simulink model "DC_Simscape_test_Sem_Graph"  (R2016a)
settings: Solver=ode15s  StartTime=0.0  StopTime=20  RelTol=1e-3
PreLoadFcn:
  | t_sim = 1;
  | T = 25;
libraries: fl_lib x16, nesl_utility x13, elec_lib x4, simulink x2
Description:
  | Schottky Barrier Diode Characteristics
  | 
  | This example shows generation of the current versus voltage curve
  | for a Schottky barrier diode. Define the vector of temperatures for
  | which to plot the characteristics by double clicking on the block
  | labeled 'Define temperatures'. Then double click on the block
  | labeled 'Generate Characteristics'. The datasheet for this device
  | gives Vf = 0.4V when If = 10mA, and Vf = 0.65V when If = 100mA.
  | The ohmic resistance is set to one over the gradient of the
  | datasheet I-V curve at higher voltages. The temperature
  | dependence is then modeled by selecting the default energy gap
  | and saturation current temperature exponent values for a Schottky
  | barrier diode. The plot produced by this test model can be used to
  | validate the implementation against the datasheet I-V plots.
  | 
  | 
  | Copyright 2008-2016 The MathWorks, Inc.
settings Model: ExtModeAutoUpdateStatusClock=off  Creator=MathWorks  LastModifiedBy=sara
settings SolverCC: ZeroCrossAlgorithm=Adaptive
settings DataIOCC: LimitDataPoints=on  SaveFormat=Array  SignalLoggingSaveFormat=ModelDataLogs  OutputOption=SpecifiedOutputTimes  OutputTimes=[0:t_sim/4000:t_sim]  Refine=5
settings OptimizationCC: ExpressionDepthLimit=2147483647  InitFltsAndDblsToZero=on
settings DebuggingCC: SaveWithParameterizedLinksMsg=none  UnderspecifiedInitializationDetection=Classic  MergeDetectMultiDrivingBlocksExec=none  SignalResolutionControl=TryResolveAllWithWarning  FcnCallInpInsideContextMsg=UseLocalSettings  StateNameClashWarn=warning
settings HardwareCC: ProdBitPerPointer=32  ProdLargestAtomicFloat=None  ProdIntDivRoundTo=Undefined  ProdEndianess=Unspecified  ProdWordSize=32  ProdHWDeviceType=32-bit Generic
settings ModelReferenceCC: PropagateSignalLabelsOutOfModel=off
settings GRTTargetCC: TargetFcnLib=ansi_tfl_tmw.mat  CombineOutputUpdateFcns=off  GRTInterface=on
settings ConfigComp: CovModelRefEnable=Off  CovSFcnEnable=off

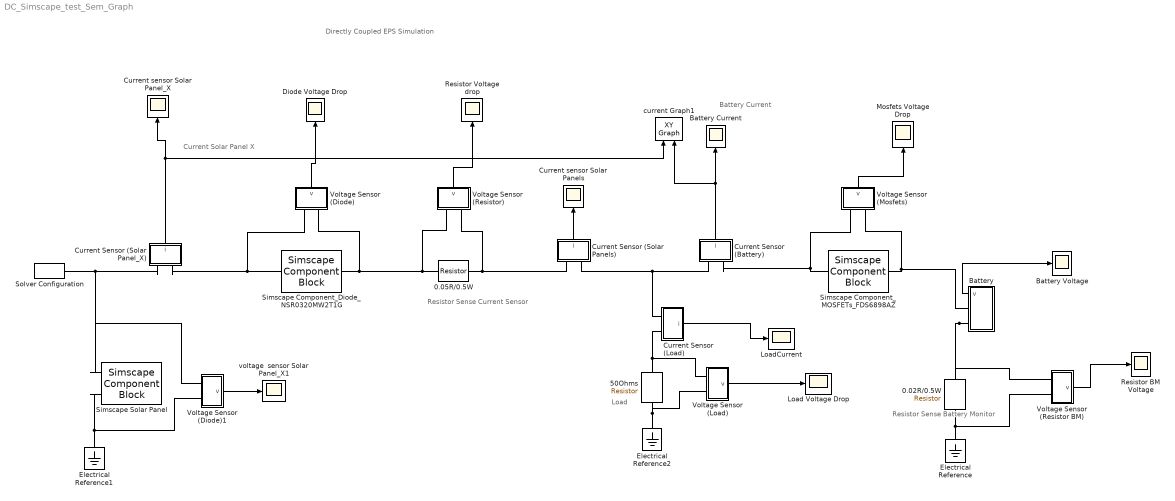
== system DC_Simscape_test_Sem_Graph ==
  note: Battery Current
  note: Resistor Sense
      | Battery Monitor
  note: Resistor Sense
      | Current Sensor
  note: Current Solar Panel X
  note: Directly Coupled EPS Simulation
  note: Load
  " Battery" : Subsystem
      settings: CopyFcn=set_param(gcb,'LinkStatus','none')
  " 0.02R/0.5W" : elec_lib/Passive Devices/Resistor  R=0.02 Ohm  R_tol=0.01  enable_R_tol=0  tol_distribution=1  nSigma=4  enable_operating_limits=0  operating_limit_action=2  max_working_voltage=100 V  power_rating=1 W  enable_faults=0  fault_action=1  R_faulted=Inf Ohm  enable_temporal_fault=0  t_fault=1 s  enable_behavioral_fault=0  max_permissible_current=1 A  t_fail_on_current=1 s  noise_mode=0  sample_time=0.001 s  repeatability=1  auto_seed=2838735261  user_seed=0  Tdevice=25 degC  alpha=0.00393 1/K  Tmeas=25 degC  thermal_mass=100 J/K  initial_temperature=25 degC  power_derating_T1=70 degC  power_derating_T2=155 degC  operating_temperature_range_vec=[ -50 150 ] degC
  " 0.05R/0.5W" : elec_lib/Passive Devices/Resistor  R=0.05 Ohm  R_tol=0.01  enable_R_tol=0  tol_distribution=1  nSigma=4  enable_operating_limits=0  operating_limit_action=2  max_working_voltage=100 V  power_rating=1 W  enable_faults=0  fault_action=1  R_faulted=Inf Ohm  enable_temporal_fault=0  t_fault=1 s  enable_behavioral_fault=0  max_permissible_current=1 A  t_fail_on_current=1 s  noise_mode=0  sample_time=0.001 s  repeatability=1  auto_seed=3991682350  user_seed=0  Tdevice=25 degC  alpha=0.00393 1/K  Tmeas=25 degC  thermal_mass=100 J/K  initial_temperature=25 degC  power_derating_T1=70 degC  power_derating_T2=155 degC  operating_temperature_range_vec=[ -50 150 ] degC
  " Current sensor Solar Panel_X" : Scope
  " Current sensor Solar Panels" : Scope
  " Resistor Voltage drop" : Scope
  50Ohms : elec_lib/Passive Devices/Resistor  R=50 Ohm  R_tol=0.01  enable_R_tol=0  tol_distribution=1  nSigma=4  enable_operating_limits=0  operating_limit_action=2  max_working_voltage=100 V  power_rating=1 W  enable_faults=0  fault_action=1  R_faulted=Inf Ohm  enable_temporal_fault=0  t_fault=1 s  enable_behavioral_fault=0  max_permissible_current=1 A  t_fail_on_current=1 s  noise_mode=0  sample_time=0.001 s  repeatability=1  auto_seed=2710425008  user_seed=0  Tdevice=25 degC  alpha=0.00393 1/K  Tmeas=25 degC  thermal_mass=100 J/K  initial_temperature=25 degC  power_derating_T1=70 degC  power_derating_T2=155 degC  operating_temperature_range_vec=[ -50 150 ] degC
  Battery Current : Scope
  Battery Voltage : Scope
  Current Sensor (Battery) : Subsystem
      settings: CopyFcn=set_param(gcb,'LinkStatus','none')
  Current Sensor (Load) : Subsystem
      settings: CopyFcn=set_param(gcb,'LinkStatus','none')
  Current Sensor (Solar Panel_X) : Subsystem
      settings: CopyFcn=set_param(gcb,'LinkStatus','none')
  Current Sensor (Solar Panels) : Subsystem
      settings: CopyFcn=set_param(gcb,'LinkStatus','none')
  Diode Voltage Drop : Scope
  Electrical Reference : fl_lib/Electrical/Electrical Elements/Electrical Reference
  Electrical Reference1 : fl_lib/Electrical/Electrical Elements/Electrical Reference
  Electrical Reference2 : fl_lib/Electrical/Electrical Elements/Electrical Reference
  Load Voltage Drop : Scope
  LoadCurrent : Scope
  Mosfets Voltage Drop : Scope
  Resistor BM Voltage : Scope
  Simscape Component_Diode_NSR0320MW2T1G : SimscapeComponentBlock  SourceFile=diode_EPS  ComponentPath=diode_EPS  ComponentVariants=diode_EPS  ComponentVariantNames=diode_EPS  ClassName=diode_EPS  SchemaVersion=1  Vt=1.38e-23 * 298 / 1.60e-19 V  R=0.0084 Ohm  n=1.00404  Is=1.3032e-6 A  i_specify=off  i_priority=None  i=1 A  v_specify=off  v_priority=None  v=0 V
      settings: CopyFcn=simscape.engine.sli.internal.componentblockcallback(gcbh,'COPY')  PreCopyFcn=simscape.engine.sli.internal.componentblockcallback(gcbh,'PRECOPY')  PreDeleteFcn=simscape.engine.sli.internal.componentblockcallback(gcbh,'PREDELETE')
      mask Type: Code produced by Embedded Systems Group - UFSC
      mask Display:
      | disp('Simscape\n\n\n')
      | disp('\n\n\ndiode_EPS');
      | color('red');
      | port_label('RConn', 1,'-');
      | port_label('LConn', 1,'+');
  Simscape Component_MOSFETs_FDS6898AZ : SimscapeComponentBlock  SourceFile=MOSFETs_EPS  ComponentPath=MOSFETs_EPS  ComponentVariants=MOSFETs_EPS  ComponentVariantNames=MOSFETs_EPS  ClassName=MOSFETs_EPS  SchemaVersion=1  Vt=1.38e-23 * 298 / 1.60e-19 V  Rsd=0.27 Ohm  Rs=0.008235 Ohm  n=1.89492  Is=1.26064e-7 A  i_specify=off  i_priority=None  i=1 A  v_specify=off  v_priority=None  v=0 V  Vr_DC_specify=off  Vr_DC_priority=None  Vr_DC=0 V  Vr_CC_specify=off  Vr_CC_priority=None  Vr_CC=0 V
      settings: CopyFcn=simscape.engine.sli.internal.componentblockcallback(gcbh,'COPY')  PreCopyFcn=simscape.engine.sli.internal.componentblockcallback(gcbh,'PRECOPY')  PreDeleteFcn=simscape.engine.sli.internal.componentblockcallback(gcbh,'PREDELETE')
      mask Type: Code produced by Embedded Systems Group - UFSC
      mask Display:
      | disp('Simscape\n\n\n')
      | disp('\n\n\nMOSFETs_EPS');
      | color('red');
      | port_label('RConn', 1,'-');
      | port_label('LConn', 1,'+');
  Simscape Solar Panel : SimscapeComponentBlock  SourceFile=simscape.solarPanel  ComponentPath=simscape.solarPanel  ComponentVariants=simscape.solarPanel  ComponentVariantNames=solarPanel  ClassName=solarPanel  SchemaVersion=1  Rs=5.59404 Ohm  Rsh=954.801 Ohm  A=2.1  Ir=2.37917e-07 A  Iph=0 A  Np=5  Ns=8  Npp=3  i_specify=off  i_priority=None  i=0 A  v_specify=off  v_priority=None  v=0 V
      settings: CopyFcn=simscape.engine.sli.internal.componentblockcallback(gcbh,'COPY')  PreCopyFcn=simscape.engine.sli.internal.componentblockcallback(gcbh,'PRECOPY')  PreDeleteFcn=simscape.engine.sli.internal.componentblockcallback(gcbh,'PREDELETE')
      mask Type: solarPanel
      mask Display: color('red');plot([0 1 1 0 0],[0 0 1 1 0]);plot([0.7,1],[1,0.7]);plot(-2,-1.75);plot(3, 1);disp('\n.ssc\nUnresolved')
  Solver Configuration : nesl_utility/Solver Configuration  PhysicalDomain=network_engine_domain  SubClassName=solver  LeftPortType=input  RightPortType=generic  Accelerate=off  Tones=[]  Harmonics=[]  SimulateNoise=off  Profile=off  UseLocalSampling=off  EnableSwitchedLinearOptims=on  FrequencyDomain=off  UseCCode=off  RelTol=0.001  AbsTol=1e-06  MinStep=1e-09  ToWorkspace=off  RevertToSquareIcSolve=off  NumHomotopyIterations=100  PhasorMode=off  PhasorModeNumHarmonics=1  OverrideAbsTol=off  DoDC=on  ResidualTolerance=1e-6  UseLocalSolver=off  LocalSolverChoice=NE_BACKWARD_EULER_ADVANCER  LocalSolverSampleTime=.001  DoFixedCost=off  MaxNonlinIter=3  MaxModeIter=2  LinearAlgebra=Sparse  DelaysMemoryBudget=1024  AutomaticFiltering=on  FilteringTimeConstant=0.001
  Voltage Sensor (Diode) : Subsystem
      settings: CopyFcn=set_param(gcb,'LinkStatus','none')
  Voltage Sensor (Diode)1 : Subsystem
      settings: CopyFcn=set_param(gcb,'LinkStatus','none')
  Voltage Sensor (Load) : Subsystem
      settings: CopyFcn=set_param(gcb,'LinkStatus','none')
  Voltage Sensor (Mosfets) : Subsystem
      settings: CopyFcn=set_param(gcb,'LinkStatus','none')
  Voltage Sensor (Resistor BM) : Subsystem
      settings: CopyFcn=set_param(gcb,'LinkStatus','none')
  "Voltage Sensor (Resistor) " : Subsystem
      settings: CopyFcn=set_param(gcb,'LinkStatus','none')
  current Graph1 : simulink/Sinks/XY Graph  xmin=-2  xmax=2  ymin=-2  ymax=2  st=-1
  voltage  sensor Solar Panel_X1 : Scope
  wires:
  Voltage Sensor (Mosfets)/1(v) -> Mosfets Voltage Drop/1
  " Battery"/1(v) -> Battery Voltage/1
  Voltage Sensor (Diode)/1(v) -> Diode Voltage Drop/1
  Current Sensor (Solar Panels)/1(i) -> " Current sensor Solar Panels"/1
  "Voltage Sensor (Resistor) "/1(v) -> " Resistor Voltage drop"/1
  Voltage Sensor (Resistor BM)/1(v) -> Resistor BM Voltage/1
  Voltage Sensor (Load)/1(v) -> Load Voltage Drop/1
  Current Sensor (Load)/1(i) -> LoadCurrent/1
  Voltage Sensor (Diode)1/1(v) -> voltage  sensor Solar Panel_X1/1
  Current Sensor (Battery)/1(i) -> current Graph1/2, Battery Current/1
  Current Sensor (Solar Panel_X)/1(i) -> current Graph1/1, " Current sensor Solar Panel_X"/1
  connections:
  Voltage Sensor (Diode)/LConn1 -- Simscape Component_Diode_NSR0320MW2T1G/LConn1 -- Current Sensor (Solar Panel_X)/LConn2
  " Battery"/RConn2 -- Voltage Sensor (Resistor BM)/LConn1 -- " 0.02R/0.5W"/LConn1
  Simscape Component_Diode_NSR0320MW2T1G/RConn1 -- "Voltage Sensor (Resistor) "/LConn1 -- " 0.05R/0.5W"/LConn1 -- Voltage Sensor (Diode)/LConn2
  Simscape Component_MOSFETs_FDS6898AZ/LConn1 -- Current Sensor (Battery)/LConn2 -- Voltage Sensor (Mosfets)/LConn1
  Current Sensor (Solar Panels)/LConn1 -- "Voltage Sensor (Resistor) "/LConn2 -- " 0.05R/0.5W"/RConn1
  Current Sensor (Solar Panel_X)/LConn1 -- Voltage Sensor (Diode)1/LConn1 -- Simscape Solar Panel/LConn1 -- Solver Configuration/RConn1
  Current Sensor (Load)/LConn1 -- Current Sensor (Solar Panels)/LConn2 -- Current Sensor (Battery)/LConn1
  Electrical Reference/LConn1 -- Voltage Sensor (Resistor BM)/LConn2 -- " 0.02R/0.5W"/RConn1
  Electrical Reference2/LConn1 -- Voltage Sensor (Load)/LConn2 -- 50Ohms/RConn1
  50Ohms/LConn1 -- Current Sensor (Load)/LConn2 -- Voltage Sensor (Load)/LConn1
  Voltage Sensor (Mosfets)/LConn2 -- " Battery"/RConn1 -- Simscape Component_MOSFETs_FDS6898AZ/RConn1
  Simscape Solar Panel/LConn2 -- Voltage Sensor (Diode)1/LConn2 -- Electrical Reference1/LConn1

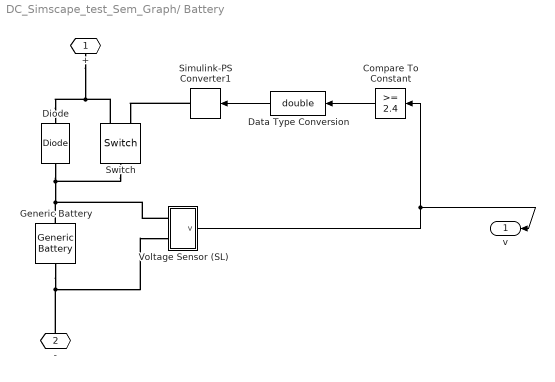
== system DC_Simscape_test_Sem_Graph/ Battery ==
  Compare To Constant : simulink/Logic and Bit Operations/Compare To Constant  relop=>=  const=2.4  OutDataTypeStr=boolean
  Data Type Conversion : DataTypeConversion  OutDataTypeStr=double
  Diode : fl_lib/Electrical/Electrical Elements/Diode  Vf=0.0001 V  Ron=0.0001 Ohm  Goff=1e-8 1/Ohm  i_specify=off  i_priority=None  i=0 A  v_specify=off  v_priority=None  v=0 V
  Generic Battery : elec_lib/Sources/Generic Battery  Vnom=3.7 V  R1=0.01 Ohm  prm_AH=2  AH=3 hr*A  AH0=1 hr*A  V1=3 V  AH1=1 hr*A  prm_R2=1  R2=2e+3 Ohm
  Simulink-PS Converter1 : nesl_utility/Simulink-PS Converter  PhysicalDomain=network_engine_domain  SubClassName=ps_input  LeftPortType=input  RightPortType=output  PseudoPeriodic=off  Frequencies=[]  NoiseDistribution=none  NoiseParameters=[]  Unit=A  AffineConversion=off  InputFiltering=off  SimscapeFilterOrder=1  InputFilterTimeConstant=.001  UdotUserProvided=0
  Switch : fl_lib/Electrical/Electrical Elements/Switch  R_closed=0.01 Ohm  G_open=1e-8 1/Ohm  Threshold=0  i_specify=off  i_priority=None  i=0 A  v_specify=off  v_priority=None  v=0 V
  Voltage Sensor (SL) : Subsystem
      settings: CopyFcn=set_param(gcb,'LinkStatus','none')
  + : PMIOPort  Port=1  Side=Right
  - : PMIOPort  Port=2  Side=Right
  v : Outport
  wires:
  Voltage Sensor (SL)/1(v) -> v/1, Compare To Constant/1
  Data Type Conversion/1 -> Simulink-PS Converter1/1
  Compare To Constant/1 -> Data Type Conversion/1
  connections:
  -/RConn1 -- Generic Battery/RConn1 -- Voltage Sensor (SL)/LConn2
  Voltage Sensor (SL)/LConn1 -- Generic Battery/LConn1 -- Diode/RConn1 -- Switch/LConn1
  Simulink-PS Converter1/RConn1 -- Switch/RConn1
  Diode/LConn1 -- Switch/RConn2 -- +/RConn1

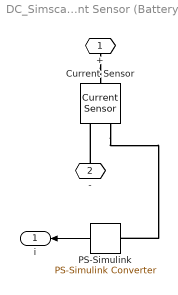
== system DC_Simscape_test_Sem_Graph/Current Sensor (Battery) ==
  Current Sensor : fl_lib/Electrical/Electrical Sensors/Current Sensor
  PS-Simulink : nesl_utility/PS-Simulink Converter  PhysicalDomain=network_engine_domain  SubClassName=ps_output  LeftPortType=input  RightPortType=output  PseudoPeriodic=off  Frequencies=[]  Unit=A  AffineConversion=off
  + : PMIOPort  Port=1  Side=Left
  - : PMIOPort  Port=2  Side=Left
  i : Outport
  wires:
  PS-Simulink/1 -> i/1
  connections:
  -/RConn1 -- Current Sensor/RConn2
  +/RConn1 -- Current Sensor/LConn1
  Current Sensor/RConn1 -- PS-Simulink/LConn1

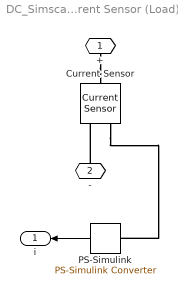
== system DC_Simscape_test_Sem_Graph/Current Sensor (Load) ==
  Current Sensor : fl_lib/Electrical/Electrical Sensors/Current Sensor
  PS-Simulink : nesl_utility/PS-Simulink Converter  PhysicalDomain=network_engine_domain  SubClassName=ps_output  LeftPortType=input  RightPortType=output  PseudoPeriodic=off  Frequencies=[]  Unit=A  AffineConversion=off
  + : PMIOPort  Port=1  Side=Left
  - : PMIOPort  Port=2  Side=Left
  i : Outport
  wires:
  PS-Simulink/1 -> i/1
  connections:
  -/RConn1 -- Current Sensor/RConn2
  +/RConn1 -- Current Sensor/LConn1
  Current Sensor/RConn1 -- PS-Simulink/LConn1

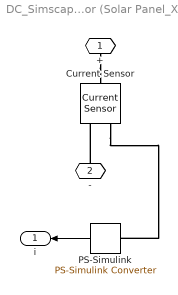
== system DC_Simscape_test_Sem_Graph/Current Sensor (Solar Panel_X) ==
  Current Sensor : fl_lib/Electrical/Electrical Sensors/Current Sensor
  PS-Simulink : nesl_utility/PS-Simulink Converter  PhysicalDomain=network_engine_domain  SubClassName=ps_output  LeftPortType=input  RightPortType=output  PseudoPeriodic=off  Frequencies=[]  Unit=A  AffineConversion=off
  + : PMIOPort  Port=1  Side=Left
  - : PMIOPort  Port=2  Side=Left
  i : Outport
  wires:
  PS-Simulink/1 -> i/1
  connections:
  -/RConn1 -- Current Sensor/RConn2
  +/RConn1 -- Current Sensor/LConn1
  Current Sensor/RConn1 -- PS-Simulink/LConn1

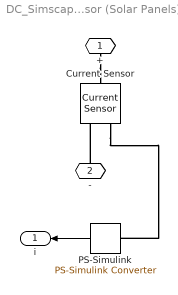
== system DC_Simscape_test_Sem_Graph/Current Sensor (Solar Panels) ==
  Current Sensor : fl_lib/Electrical/Electrical Sensors/Current Sensor
  PS-Simulink : nesl_utility/PS-Simulink Converter  PhysicalDomain=network_engine_domain  SubClassName=ps_output  LeftPortType=input  RightPortType=output  PseudoPeriodic=off  Frequencies=[]  Unit=A  AffineConversion=off
  + : PMIOPort  Port=1  Side=Left
  - : PMIOPort  Port=2  Side=Left
  i : Outport
  wires:
  PS-Simulink/1 -> i/1
  connections:
  -/RConn1 -- Current Sensor/RConn2
  +/RConn1 -- Current Sensor/LConn1
  Current Sensor/RConn1 -- PS-Simulink/LConn1

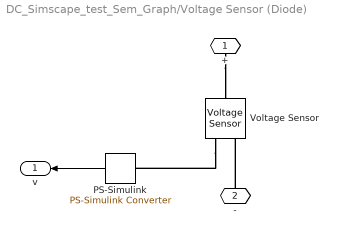
== system DC_Simscape_test_Sem_Graph/Voltage Sensor (Diode) ==
  PS-Simulink : nesl_utility/PS-Simulink Converter  PhysicalDomain=network_engine_domain  SubClassName=ps_output  LeftPortType=input  RightPortType=output  PseudoPeriodic=off  Frequencies=[]  Unit=V  AffineConversion=off
  Voltage Sensor : fl_lib/Electrical/Electrical Sensors/Voltage Sensor
  + : PMIOPort  Port=1  Side=Left
  - : PMIOPort  Port=2  Side=Left
  v : Outport
  wires:
  PS-Simulink/1 -> v/1
  connections:
  -/RConn1 -- Voltage Sensor/RConn2
  +/RConn1 -- Voltage Sensor/LConn1
  Voltage Sensor/RConn1 -- PS-Simulink/LConn1

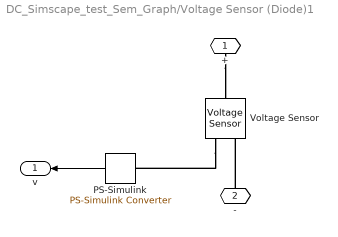
== system DC_Simscape_test_Sem_Graph/Voltage Sensor (Diode)1 ==
  PS-Simulink : nesl_utility/PS-Simulink Converter  PhysicalDomain=network_engine_domain  SubClassName=ps_output  LeftPortType=input  RightPortType=output  PseudoPeriodic=off  Frequencies=[]  Unit=V  AffineConversion=off
  Voltage Sensor : fl_lib/Electrical/Electrical Sensors/Voltage Sensor
  + : PMIOPort  Port=1  Side=Left
  - : PMIOPort  Port=2  Side=Left
  v : Outport
  wires:
  PS-Simulink/1 -> v/1
  connections:
  -/RConn1 -- Voltage Sensor/RConn2
  +/RConn1 -- Voltage Sensor/LConn1
  Voltage Sensor/RConn1 -- PS-Simulink/LConn1

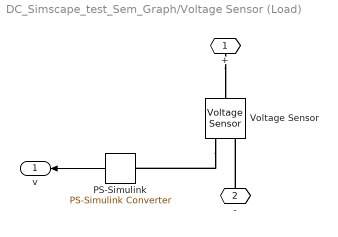
== system DC_Simscape_test_Sem_Graph/Voltage Sensor (Load) ==
  PS-Simulink : nesl_utility/PS-Simulink Converter  PhysicalDomain=network_engine_domain  SubClassName=ps_output  LeftPortType=input  RightPortType=output  PseudoPeriodic=off  Frequencies=[]  Unit=V  AffineConversion=off
  Voltage Sensor : fl_lib/Electrical/Electrical Sensors/Voltage Sensor
  + : PMIOPort  Port=1  Side=Left
  - : PMIOPort  Port=2  Side=Left
  v : Outport
  wires:
  PS-Simulink/1 -> v/1
  connections:
  -/RConn1 -- Voltage Sensor/RConn2
  +/RConn1 -- Voltage Sensor/LConn1
  Voltage Sensor/RConn1 -- PS-Simulink/LConn1

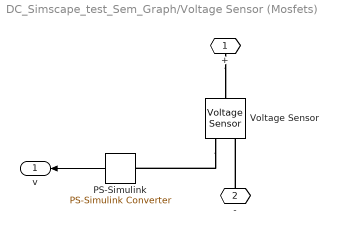
== system DC_Simscape_test_Sem_Graph/Voltage Sensor (Mosfets) ==
  PS-Simulink : nesl_utility/PS-Simulink Converter  PhysicalDomain=network_engine_domain  SubClassName=ps_output  LeftPortType=input  RightPortType=output  PseudoPeriodic=off  Frequencies=[]  Unit=V  AffineConversion=off
  Voltage Sensor : fl_lib/Electrical/Electrical Sensors/Voltage Sensor
  + : PMIOPort  Port=1  Side=Left
  - : PMIOPort  Port=2  Side=Left
  v : Outport
  wires:
  PS-Simulink/1 -> v/1
  connections:
  -/RConn1 -- Voltage Sensor/RConn2
  +/RConn1 -- Voltage Sensor/LConn1
  Voltage Sensor/RConn1 -- PS-Simulink/LConn1

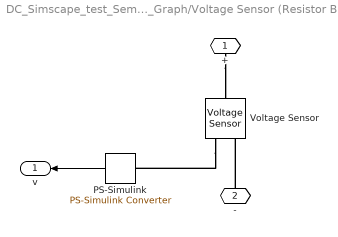
== system DC_Simscape_test_Sem_Graph/Voltage Sensor (Resistor BM) ==
  PS-Simulink : nesl_utility/PS-Simulink Converter  PhysicalDomain=network_engine_domain  SubClassName=ps_output  LeftPortType=input  RightPortType=output  PseudoPeriodic=off  Frequencies=[]  Unit=V  AffineConversion=off
  Voltage Sensor : fl_lib/Electrical/Electrical Sensors/Voltage Sensor
  + : PMIOPort  Port=1  Side=Left
  - : PMIOPort  Port=2  Side=Left
  v : Outport
  wires:
  PS-Simulink/1 -> v/1
  connections:
  -/RConn1 -- Voltage Sensor/RConn2
  +/RConn1 -- Voltage Sensor/LConn1
  Voltage Sensor/RConn1 -- PS-Simulink/LConn1

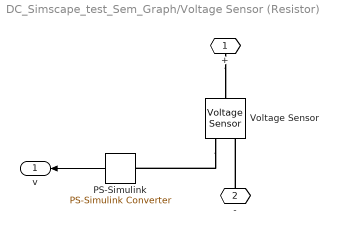
== system DC_Simscape_test_Sem_Graph/Voltage Sensor (Resistor)  ==
  PS-Simulink : nesl_utility/PS-Simulink Converter  PhysicalDomain=network_engine_domain  SubClassName=ps_output  LeftPortType=input  RightPortType=output  PseudoPeriodic=off  Frequencies=[]  Unit=V  AffineConversion=off
  Voltage Sensor : fl_lib/Electrical/Electrical Sensors/Voltage Sensor
  + : PMIOPort  Port=1  Side=Left
  - : PMIOPort  Port=2  Side=Left
  v : Outport
  wires:
  PS-Simulink/1 -> v/1
  connections:
  -/RConn1 -- Voltage Sensor/RConn2
  +/RConn1 -- Voltage Sensor/LConn1
  Voltage Sensor/RConn1 -- PS-Simulink/LConn1

== system DC_Simscape_test_Sem_Graph/ Battery/Voltage Sensor (SL) ==
  PS-Simulink : nesl_utility/PS-Simulink Converter  PhysicalDomain=network_engine_domain  SubClassName=ps_output  LeftPortType=input  RightPortType=output  PseudoPeriodic=off  Frequencies=[]  Unit=V  AffineConversion=off
  Voltage Sensor : fl_lib/Electrical/Electrical Sensors/Voltage Sensor
  + : PMIOPort  Port=1  Side=Left
  - : PMIOPort  Port=2  Side=Left
  v : Outport
  wires:
  PS-Simulink/1 -> v/1
  connections:
  -/RConn1 -- Voltage Sensor/RConn2
  +/RConn1 -- Voltage Sensor/LConn1
  Voltage Sensor/RConn1 -- PS-Simulink/LConn1
